simulink model "task_07_simulink"  (R2024b)
settings: Solver=VariableStepAuto  StartTime=0.0  StopTime=10.0  RelTol=1e-3
libraries: cstblocks x2
settings Model: Creator=jx2004  LastModifiedBy=jx2004

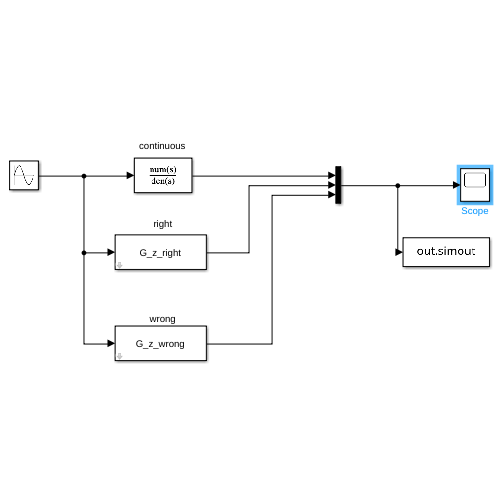
[thumbnail: Simulink's stored preview of the top-level diagram]
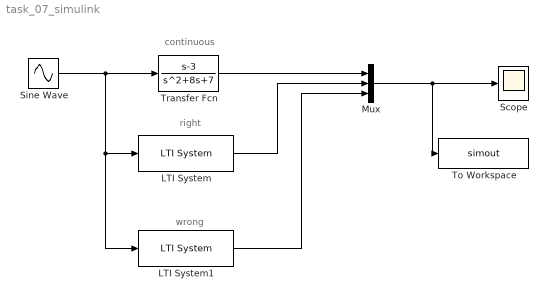
== system task_07_simulink ==
  note: continuous
  note: right
  note: wrong
  LTI System : cstblocks/LTI System  sys=G_z_right  IC=[]  PadeOrder=0
  LTI System1 : cstblocks/LTI System  sys=G_z_wrong  IC=[]  PadeOrder=0
  Mux : Mux  Inputs=3
  Scope : Scope
  Sine Wave : Sin  SampleTime=0
  To Workspace : ToWorkspace  VariableName=simout  SaveFormat=Timeseries  SampleTime=-1
  Transfer Fcn : TransferFcn  Numerator=[1 -3]  Denominator=[1 8 7]
  wires:
  Transfer Fcn/1 -> Mux/1
  LTI System/1 -> Mux/2
  LTI System1/1 -> Mux/3
  Sine Wave/1 -> LTI System1/1, LTI System/1, Transfer Fcn/1
  Mux/1 -> To Workspace/1, Scope/1
